simulink model "MSDsystem_temp"  (R2023b)
settings: Solver=ode4  StartTime=0.0  StopTime=25  FixedStep=1e-2  RelTol=1e-3  AbsTol=1e-6
values from neighbouring files (symbols this model uses):
  b = 2    [Lecture_1_Exercises.m]
  k = 2    [Lecture_1_Exercises.m]
  m = 1    [Lecture_1_Exercises.m]
settings Model: Creator=jerome  LastModifiedBy=Therkelsen
settings SolverCC: AutoScaleAbsTol=off  AlgebraicLoopSolver=TrustRegion
settings DataIOCC: SaveFormat=Array  SignalLoggingSaveFormat=ModelDataLogs  ReturnWorkspaceOutputs=off
settings OptimizationCC: BlockReduction=off  BooleanDataType=off  ExpressionDepthLimit=2147483647  InitFltsAndDblsToZero=on  LifeSpan=inf
settings DebuggingCC: SaveWithParameterizedLinksMsg=none  UnderspecifiedInitializationDetection=Classic  MergeDetectMultiDrivingBlocksExec=none  SignalResolutionControl=TryResolveAllWithWarning  MultiTaskDSMMsg=warning  MultiTaskCondExecSysMsg=none  FcnCallInpInsideContextMsg=warning  UnconnectedInputMsg=warning  UnconnectedOutputMsg=warning  UnconnectedLineMsg=warning  StateNameClashWarn=warning  SFUnexpectedBacktrackingDiag=warning  SFNoUnconditionalDefaultTransitionDiag=warning  SFExecutionAtInitializationDiag=none  ArithmeticOperatorsInVariantConditions=warning
settings HardwareCC: ProdBitPerPointer=32  ProdBitPerSizeT=32  ProdBitPerPtrDiffT=32  ProdLargestAtomicFloat=None  ProdIntDivRoundTo=Undefined  ProdEndianess=Unspecified  ProdWordSize=32  ProdHWDeviceType=32-bit Generic  TargetUnknown=on
settings ModelReferenceCC: EnableRefExpFcnMdlSchedulingChecks=on  PropagateSignalLabelsOutOfModel=off
settings SFSimCC: SimUseLocalCustomCode=off  CustomCodeUndefinedFunction=UseInterfaceOnly
settings RTWCC: RTWUseLocalCustomCode=off  DLArmComputeVersion=19.05
settings CodeAppCC: StateflowObjectComments=on
settings GRTTargetCC: TargetFcnLib=ansi_tfl_tmw.mat  TargetLangStandard=C89/C90 (ANSI)  ModelReferenceCompliant=off  CombineOutputUpdateFcns=off  MatFileLogging=off  GRTInterface=on
settings ConfigComp: CovMetricSettings=dw  CovSaveCumulativeToWorkspaceVar=on  CovSaveSingleToWorkspaceVar=on  CovExternalEMLEnable=off

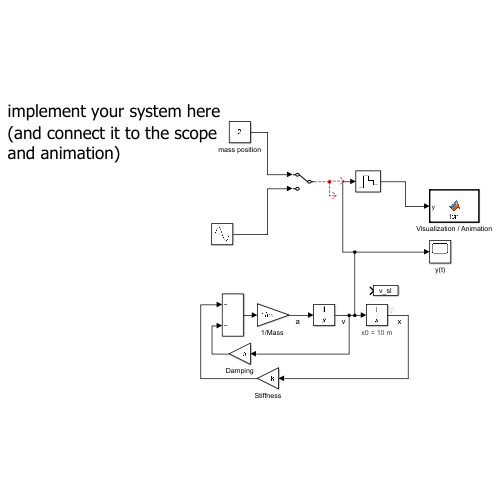
[thumbnail: Simulink's stored preview of the top-level diagram]
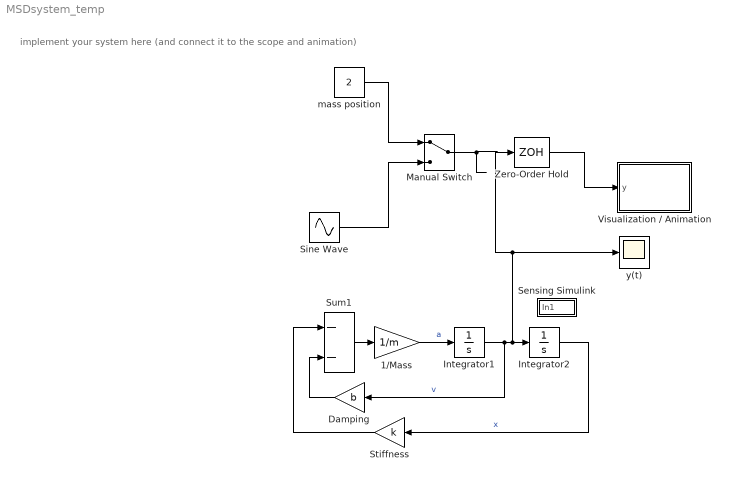
== system MSDsystem_temp ==
  note: implement your system here
      | (and connect it to the scope and animation)
  "1/Mass " : Gain  Gain=1/m  SaturateOnIntegerOverflow=on  OutDataTypeStr=Inherit: Same as input  ParamDataTypeStr=Inherit: Same as input
  Damping : Gain  Gain=b  SaturateOnIntegerOverflow=on  OutDataTypeStr=Inherit: Same as input  ParamDataTypeStr=Inherit: Same as input
  Integrator1 : Integrator
  Integrator2 : Integrator  InitialCondition=10
      settings: AttributesFormatString=x0 = %<InitialCondition> m
  Manual Switch : ManualSwitch
  Sensing Simulink : Subsystem
      mask Display: disp('v_sl')
  Sine Wave : Sin  Amplitude=10  Bias=10  SampleTime=0
  Stiffness : Gain  Gain=k  SaturateOnIntegerOverflow=on  OutDataTypeStr=Inherit: Same as input  ParamDataTypeStr=Inherit: Same as input
  Sum1 : Sum  Inputs=--  InputSameDT=on  SaturateOnIntegerOverflow=on  OutDataTypeStr=Inherit: Same as first input
  Visualization / Animation : MATLAB Function  TreatAsAtomicUnit=on
  Zero-Order Hold : ZeroOrderHold  SampleTime=0.1
  mass position : Constant  Value=2
  y(t) : Scope
  wires:
  Zero-Order Hold/1 -> Visualization / Animation/1(y)
  Manual Switch/1 -> ?
  mass position/1 -> Manual Switch/1
  Sine Wave/1 -> Manual Switch/2
  Sum1/1 -> "1/Mass "/1
  Integrator1/1 -> y(t)/1, Zero-Order Hold/1, Integrator2/1, Damping/1  "v"
  Integrator2/1 -> Stiffness/1  "x"
  "1/Mass "/1 -> Integrator1/1  "a"
  Damping/1 -> Sum1/2
  Stiffness/1 -> Sum1/1

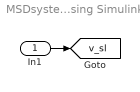
== system MSDsystem_temp/Sensing Simulink ==
  In1 : Inport
  tag scope: v_sl=global
  wires:
  In1/1 -> [v_sl]

== matlab function MSDsystem_temp/Visualization // Animation ==
  data: y input
function fcn(y)


% the mass
    Xmass = [ 5 ; 5 ; -5 ; -5 ; 5 ] + y;
    Ymass = [ -5 ; 5 ; 5 ; -5 ; -5]; 

% the spring
    Xspring = [ 0 ; 4 ; 6 ; 10 ; 14 ; 18 ; 20 ; 24 ]/24*(y+24) - 29;
    Yspring = [ 0 ; 0 ; 3 ; -3 ; 3 ; -3 ; 0 ; 0 ];

% to be able to use 'fill' even though the function is not supported for code generation
% see https://se.mathworks.com/help/simulink/slref/coder.extrinsic.html
coder.extrinsic('fill'); 

% draw the mass of the MSD system
fill(Xmass,Ymass,'r');

hold on
% draw the spring
plot(Xspring,Yspring,'b','Linewidth',3);

% draw misc
plot([-29 -29],[-10 10],'k','Linewidth',3); %draw a thick line on the left
plot([0 0],[-10 -7],'k','Linewidth',2);  % draw a thin line at position x = 0

hold off

axis([-40 40 -10 10]);
title('Mass-Spring-Damper system', 'FontSize',20);
axis equal;
grid on;

drawnow;
